simulink model "final_project"  (R2021a)
settings: Solver=FixedStepAuto  StartTime=0.0  StopTime=30  RelTol=1e-3
InitFcn:
  | load('BusDefinitions.mat')
values from neighbouring files (symbols this model uses):
  A_a_dis = [1  -0.0479044950468; 0  1]    [RSdata_Kalman.mat]
  A_e_dis = [1  0.0479044950468; 0  1]    [RSdata_Kalman.mat]
  A_t_dis = [1  0.00488821378028; 0  1]    [RSdata_Kalman.mat]
  B_a_dis = [-0.000119761237617 0.005]    [RSdata_Kalman.mat]
  B_e_dis = [0.000119761237617 0.005]    [RSdata_Kalman.mat]
  B_t_dis = [1.22205344507e-05 0.005]    [RSdata_Kalman.mat]
  C_a_dis = [1  0; 0  1]    [RSdata_Kalman.mat]
  C_e_dis = [1  0; 0  1]    [RSdata_Kalman.mat]
  C_t_dis = [1 0]    [RSdata_Kalman.mat]
  F_aileron = 5.76146350631e-05    [RSdata_Kalman.mat]
  F_elevator = -6.47120901071e-05    [RSdata_Kalman.mat]
  F_rudder = 0.000879878480451    [RSdata_Kalman.mat]
  F_throttle = -0.417330356587    [RSdata_Kalman.mat]
  g = 9.8    [RSdata_Kalman.mat]
  K_A = [5.76146350631e-05 0.000978114789418 0.000483]    [RSdata_Kalman.mat]
  K_E = [-6.47120901071e-05 0.00109860719101 0.0005425]    [RSdata_Kalman.mat]
  K_R = [0.000879878480451 0.00075]    [RSdata_Kalman.mat]
  K_T = [-0.417330356587 -0.34]    [RSdata_Kalman.mat]
  Kappa = 1    [RSdata_Kalman.mat]
  m = 0.068    [RSdata_Kalman.mat]
  M = [2.03476350051e-06 9.69056117119e-08 9.69056117119e-08 -1.05662818468e-08 2.03476350051e-06 -9.69056117119e-08 9.69056117119e-08 1.05662818468e-08 2.03476350051e-06 -9.69056117119e-08 -9.69056117119e-08 -1.05662818468e-08 ... (16 elements, 4x4)]    [RSdata_Kalman.mat]
  R_t = 0.00678306479724    [RSdata_Kalman.mat]
undefined symbols (not defined in the file or in its folder): codertarget, Discrete, Time
libraries: simulink x8, ctrlSharedLib x3
settings Model: ExtModeTrigDuration=80  Creator=tomwh  LastModifiedBy=Liza
settings SolverCC: AlgebraicLoopSolver=TrustRegion
settings OptimizationCC: EnhancedBackFolding=on  PassReuseOutputArgsAs=Individual arguments  ZeroExternalMemoryAtStartup=off  ZeroInternalMemoryAtStartup=off  MaxStackSize=64  OptimizeBlockOrder=speed  DifferentSizesBufferReuse=on  OptimizationCustomize=off  EfficientTunableParamExpr=on
settings DebuggingCC: ParameterTunabilityLossMsg=error  SFMachineParentedDataDiag=warning  ArithmeticOperatorsInVariantConditions=warning
settings HardwareCC: ProdBitPerPointer=32  ProdBitPerSizeT=32  ProdBitPerPtrDiffT=32  ProdLargestAtomicInteger=Long  ProdWordSize=32  ProdHWDeviceType=ARM Compatible->ARM 9  UseEmbeddedCoderFeatures=off
settings SFSimCC: SimUseLocalCustomCode=off  MATLABDynamicMemAlloc=off
settings RTWCC: SystemTargetFile=ert.tlc  HardwareBoard=PARROT Mambo  TemplateMakefile=ert_default_tmf  GenerateReport=on  RTWUseLocalCustomCode=off  Toolchain=Sourcery G++ Lite GNU Toolchain for Drones  LaunchReport=on
settings CodeAppCC: ForceParamTrailComments=on  IgnoreCustomStorageClasses=off  OperatorAnnotations=on  SimulinkDataObjDesc=on  SFDataObjDesc=on  InsertBlockDesc=on
settings ERTTargetCC: MatFileLogging=on  SupportNonInlinedSFcns=on

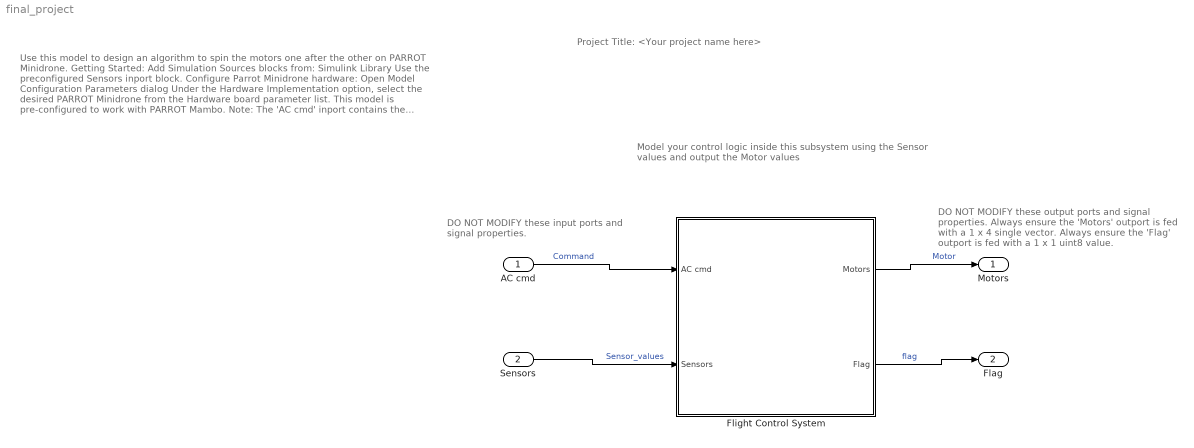
== system final_project ==
  note: Model your control logic inside this subsystem
      | using the Sensor values and output the
      | Motor values
  note: DO NOT MODIFY these output ports
      | and signal properties.
      |
      |
      |
      | Always ensure the 'Motors' outport
      | is fed with a 1 x 4 single vector.
      |
      |
      |
      |
      |
      | Always ensure the 'Flag' outport is
      | fed with a 1 x 1 uint8 value.
  note: DO NOT MODIFY these input
      | ports and signal properties.
  note: Use this model to design an algorithm to spin the motors one
      | after the other on PARROT Minidrone.
      |
      | Getting Started:
      |
      | Add Simulation Sources blocks from:
      | Simulink Library
      | Use the preconfigured Sensors inport block.
      |
      | Configure Parrot Minidrone hardware:
      |
      | Open Model Configuration Parameters dialog
      |
      | Under the Hardware Implementation option, select the desired
      | PARROT Minidrone from the Hardware board parameter list.
      |
      | This model is pre-configured to work with PARROT Mambo.
      |
      | Note:
      |
      | The 'AC cmd' inport contains the position and orientation
      | reference signals information.
      | The 'Sensors' inport contains data from accelerometer,
      | gyroscope, ultrasonic, pressure and optical flow data.
      | The 'Flag' outport can be used to model an error condition
      | which stops the drone.
      | The 'Motors' outport is fed with the speed values of the 4 motors.
      | Learn more:
      |
      | Simulink Subsystem
      | Simulink Buses
  note: Project Title: <Your project name here>
  AC cmd : Inport  OutDataTypeStr=Bus: CommandBus  BusOutputAsStruct=on
  Sensors : Inport  Port=2  OutDataTypeStr=Bus: SensorsBus  BusOutputAsStruct=on
  Flight Control System : Subsystem  InitFcn=codertarget.parrot.internal.fcsSubsystemCallback(gcb);
  Motors : Outport  OutDataTypeStr=single  PortDimensions=[1 4]  VectorParamsAs1DForOutWhenUnconnected=off
  Flag : Outport  Port=2  OutDataTypeStr=uint8  PortDimensions=1  VectorParamsAs1DForOutWhenUnconnected=off
  wires:
  Flight Control System/1(Motors) -> Motors/1  "Motor"
  AC cmd/1 -> Flight Control System/1(AC cmd)  "Command"
  Sensors/1 -> Flight Control System/2(Sensors)  "Sensor_values"
  Flight Control System/2(Flag) -> Flag/1  "flag"

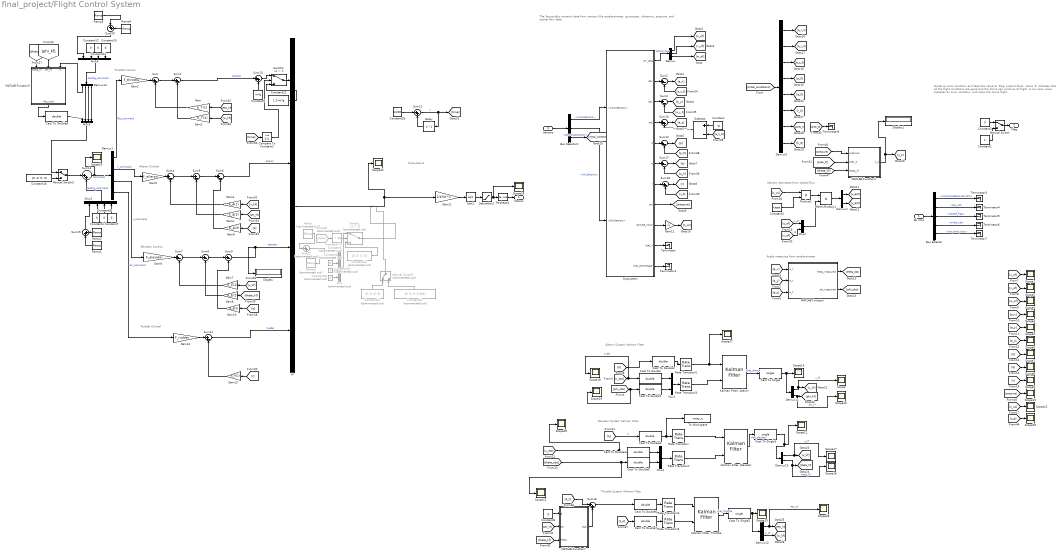
== system final_project/Flight Control System ==
  note: Subsystem1
  note: Angle measures from accelerometer
  note: Velocity estimates from optical flow
  note: Model an error condition and feed the value to 'Flag' outport block.
      | Value '0' indicates that all the flight conditions are good and the drone
      | can continue its flight.
      | A non-zero value indicates an error condition, and stops the drone
      | flight.
  note: The SensorsBus contains data from sensors like
      | accelerometer, gyroscope, ultrasonic, pressure,
      | and optical flow data.
  note: Throttle System Kalman Filter
  note: Elevator System Kalman Filter
  note: Aileron System Kalman Filter
  note: Elevator Control
  note: Aileron Control
  note: Throttle Control
  note: Rudder Control
  AC cmd : Inport
  Sensors : Inport  Port=2
  Bus Selector : BusSelector  OutputSignals=controlModePosVSOrient,pos_ref,takeoff_flag,orient_ref,live_time_ticks
  Bus Selector1 : BusSelector  OutputSignals=VisionSensors,HALSensors,SensorCalibration
  Cast To Double{,1..8} (9 alike) : DataTypeConversion  OutDataTypeStr=double
  Cast To Single : DataTypeConversion  OutDataTypeStr=single
  Cast To Single1 : DataTypeConversion  OutDataTypeStr=single
  Cast To Single2 : DataTypeConversion  OutDataTypeStr=single
  Compare To Constant1 : simulink/Logic and Bit Operations/Compare To Constant  Commented=on  relop=<  const=15  OutDataTypeStr=boolean
  Compare To Constant2 : simulink/Logic and Bit Operations/Compare To Constant  relop=>=  const=0.4  OutDataTypeStr=boolean
  Constant : Constant  Value=-g
  Constant1 : Constant  OutDataTypeStr=uint8
  Constant10 : Constant  Commented=on  Value=[0; 0; 0; 0.004]
  Constant11 : Constant  Commented=on  Value=[0; 0; 0; 0]
  Constant{4,6..7,12..13,15} (6 alike) : Constant  Value=0
  Constant14 : Constant  Commented=on  Value=[0; 0; 0; 0]
  Constant16 : Constant  Value=[0; 0; 0; 0]
  Constant18 : Constant  Value=1/200
  Constant19 : Constant  Commented=on  Value=0
  Constant2 : Constant  Value=0  OutDataTypeStr=uint8
  Constant20 : Constant  Commented=on  Value=0
  Constant21 : Constant  Value=1.1*m*g
  Constant3 : Constant  Value=Kappa
  Constant5 : Constant  Value=m*g
  Constant8 : Constant  Value=g
  Constant9 : Constant  Commented=on  Value=0
  Delay : Delay  DelayLength=1  SampleTime=1/200
  Demux : Demux  Outputs=3
  Demux1 : Demux
  Demux{2,10..12} (4 alike) : Demux  Outputs=2
  Demux14 : Demux
  Demux3 : Demux  Outputs=8
  Display : Display
  Display1 : Display
  From49 : From  Commented=on  GotoTag=time
  Gain : Gain  Gain=K_T(1)
  Gain1 : Gain  Gain=K_T(2)
  Gain10 : Gain  Gain=K_E(3)
  Gain11 : Gain  Gain=1/4*M  Multiplication=Matrix(K*u)
  Gain12 : Gain  Gain=-1
  Gain13 : Gain  Gain=K_R(2)
  Gain14 : Gain  Gain=F_rudder
  Gain2 : Gain  Gain=F_throttle
  Gain3 : Gain  Gain=K_A(1)
  Gain4 : Gain  Gain=K_A(2)
  Gain5 : Gain  Gain=F_aileron
  Gain6 : Gain  Gain=K_A(3)
  Gain7 : Gain  Gain=K_E(1)
  Gain8 : Gain  Gain=K_E(2)
  Gain9 : Gain  Gain=F_elevator
  "Kalman Filter, Aileron" : ctrlSharedLib/Kalman Filter  TimeDomain=Discrete-Time  UseCurrentEstimator=on  ModelSource=Individual A, B, C, D matrices  ModelSourceVariable=ss(0.95,1,1,0,1)  A=A_a_dis  B=B_a_dis  C=C_a_dis  D=0  NumberOfStates=1  NumberOfInputs=1  NumberOfOutputs=1  InitialEstimateSource=Dialog  X0=0  P0=10  UseK=off  UseGH=off  NumberOfProcessNoiseInputs=1  G=1  TimeInvariantG=on  H=0  TimeInvariantH=on  Q=Q_a_dis  TimeInvariantQ=on  R=eye(2)  TimeInvariantR=on  N=0  TimeInvariantN=on  AddInputPort=on  AddEnablePort=off  OutputEstimatedY=off  OutputP=off  Ts=1/200
  "Kalman Filter, Elevator" : ctrlSharedLib/Kalman Filter  TimeDomain=Discrete-Time  UseCurrentEstimator=on  ModelSource=Individual A, B, C, D matrices  ModelSourceVariable=ss(0.95,1,1,0,1)  A=A_e_dis  B=B_e_dis  C=C_e_dis  D=0  NumberOfStates=1  NumberOfInputs=1  NumberOfOutputs=1  InitialEstimateSource=Dialog  X0=0  P0=10  UseK=off  UseGH=off  NumberOfProcessNoiseInputs=1  G=1  TimeInvariantG=on  H=0  TimeInvariantH=on  Q=Q_e_dis  TimeInvariantQ=on  R=[1/100 0; 0 1/25]  TimeInvariantR=on  N=0  TimeInvariantN=on  AddInputPort=on  AddEnablePort=off  OutputEstimatedY=off  OutputP=off  Ts=1/200
  "Kalman Filter, Throttle" : ctrlSharedLib/Kalman Filter  TimeDomain=Discrete-Time  UseCurrentEstimator=on  ModelSource=Individual A, B, C, D matrices  ModelSourceVariable=ss(0.95,1,1,0,1)  A=A_t_dis  B=B_t_dis  C=C_t_dis  D=0  NumberOfStates=1  NumberOfInputs=1  NumberOfOutputs=1  InitialEstimateSource=Dialog  X0=0  P0=10  UseK=off  UseGH=off  NumberOfProcessNoiseInputs=1  G=1  TimeInvariantG=on  H=0  TimeInvariantH=on  Q=Q_t_dis  TimeInvariantQ=on  R=R_t  TimeInvariantR=on  N=0  TimeInvariantN=on  AddInputPort=on  AddEnablePort=off  OutputEstimatedY=off  OutputP=off  Ts=1/200
  MATLAB Function : MATLAB Function  TreatAsAtomicUnit=on
  MATLAB Function1 : MATLAB Function  TreatAsAtomicUnit=on
  MATLAB Function3 : MATLAB Function  TreatAsAtomicUnit=on
  MATLAB Function7 : MATLAB Function  TreatAsAtomicUnit=on
  Manual Switch : ManualSwitch
  Manual Switch2 : ManualSwitch  Commented=on
  Manual Switch3 : ManualSwitch
  MatrixMultiply1 : Product
  Mux : Mux  Commented=on
  Mux1 : Mux  Inputs=2
  Mux2 : Mux  Inputs=2
  Mux3 : Mux
  Mux4 : Mux  Inputs=2
  Mux5 : Mux
  Mux6 : Mux
  Product1 : Product
  Ramp : simulink/Sources/Ramp  Commented=on  slope=m*g/5  start=5  InitialOutput=0
  Ramp1 : simulink/Sources/Ramp  slope=-.2  start=30  InitialOutput=0
  Ramp2 : simulink/Sources/Ramp  slope=.2  start=25  InitialOutput=0
  Ramp3 : simulink/Sources/Ramp  slope=-.2  start=5  InitialOutput=0
  Ramp4 : simulink/Sources/Ramp  slope=.2  start=10  InitialOutput=0
  Ramp5 : simulink/Sources/Ramp  Commented=on  slope=-m*g/5  start=10  InitialOutput=0
  Rate Transition{,1..5} (6 alike) : RateTransition  OutPortSampleTime=dt
  Reshape1 : Reshape  OutputDimensionality=Customize  OutputDimensions=[1,4]
  Saturation1 : Saturate  UpperLimit=500  LowerLimit=0  OutDataTypeStr=single
  Scope{,1..27} (28 alike) : Scope
  Sqrt1 : Sqrt  SaturateOnIntegerOverflow=on
  Subsystem : Subsystem
  Subtract : Sum  Inputs=+-
  Sum{,1..9,11..12,17..18} (14 alike) : Sum  Inputs=|+-
  Sum{10,13..16,20..21} (7 alike) : Sum  Inputs=|++
  Sum22 : Sum  Commented=on  Inputs=|++
  Switch1 : Switch  Commented=on  Criteria=u2 > Threshold
  Switch2 : Switch  Criteria=u2 > Threshold
  Terminator{,1,3..8} (8 alike) : Terminator
  To Workspace : ToWorkspace  VariableName=noisy_q  SaveFormat=Structure With Time  SampleTime=-1
  W : Mux
  Motors : Outport  VectorParamsAs1DForOutWhenUnconnected=off
  Flag : Outport  Port=2  VectorParamsAs1DForOutWhenUnconnected=off
  wires:
  AC cmd/1 -> Bus Selector/1
  Bus Selector/1 -> Terminator3/1  "<controlModePosVSOrient>"
  Bus Selector/2 -> Terminator4/1  "<pos_ref>"
  Bus Selector/3 -> Terminator5/1  "<takeoff_flag>"
  Bus Selector/4 -> Terminator6/1  "<orient_ref>"
  Bus Selector/5 -> Terminator7/1  "<live_time_ticks>"
  Manual Switch/1 -> Flag/1
  Bus Selector1/1 -> Subsystem/1(<VisionSensors>)  "<VisionSensors>"
  Bus Selector1/3 -> [initial_conditions]  "<SensorCalibration>"
  Sensors/1 -> Bus Selector1/1
  Bus Selector1/2 -> Subsystem/2(<HALSensors>)  "<HALSensors>"
  Subsystem/10(vbat_V) -> Terminator/1
  Subsystem/11(vbat_percentage) -> Terminator1/1
  Subsystem/1(OF_data) -> Demux/1  "optical_flow"
  Demux/1 -> [u_of]
  Demux/2 -> [v_of]
  Demux/3 -> [w_of]
  Subsystem/8(prs) -> [pressure]
  [u_of] -> Scope1/1
  [v_of] -> Scope2/1
  [w_of] -> Scope3/1
  [a_x] -> Scope4/1
  [a_y] -> Scope5/1
  [a_z] -> Scope6/1
  [p] -> Scope7/1
  [q] -> Scope8/1
  [r] -> Scope9/1
  [pressure] -> Scope12/1
  [z_us] -> Scope13/1
  Mux2/1 -> MatrixMultiply1/2
  Product1/1 -> MatrixMultiply1/1
  [v_of] -> Mux2/2  "v_of"
  Demux2/2 -> [v_est]
  MatrixMultiply1/1 -> Demux2/1
  Demux2/1 -> [u_est]
  Constant3/1 -> Product1/2
  [u_of] -> Mux2/1  "u_of"
  [z_us] -> Product1/1
  [a_z] -> MATLAB Function/3(a_z)
  [a_x] -> MATLAB Function/1(a_x)
  [a_y] -> MATLAB Function/2(a_y)
  MATLAB Function/1(theta_measured) -> [theta_obs]
  MATLAB Function/2(phi_measured) -> [phi_obs]
  Constant2/1 -> Manual Switch/1
  Constant1/1 -> Manual Switch/2
  Sqrt1/1 -> Saturation1/1
  "Kalman Filter, Throttle"/1 -> Cast To Single2/1  "xhat_throttle"
  [v_est] -> Scope18/1, Cast To Double/1  "v_est"
  Mux4/1 -> Rate Transition1/1
  Demux12/1 -> Scope26/1, [Pbz_kf]  "Pbz_kf"
  Cast To Double2/1 -> Rate Transition2/1
  Cast To Single/1 -> Demux11/1, Scope14/1
  Cast To Double4/1 -> Mux4/1
  Demux12/2 -> [w_kf]  "w_kf"
  Demux10/1 -> Scope17/1, [u_kf]  "u_kf"
  Mux1/1 -> Rate Transition3/1
  Rate Transition/1 -> "Kalman Filter, Elevator"/1
  [phi_obs] -> Scope19/1, Cast To Double1/1
  Rate Transition5/1 -> "Kalman Filter, Throttle"/2
  "Kalman Filter, Aileron"/1 -> Cast To Single/1  "xhat_aileron"
  Demux11/2 -> Scope10/1, [phi_kf]  "phi_kf"
  Sum16/1 -> Cast To Double6/1
  Rate Transition3/1 -> "Kalman Filter, Aileron"/2
  Cast To Double7/1 -> Rate Transition5/1
  Rate Transition2/1 -> Scope27/1, "Kalman Filter, Aileron"/1
  Demux10/2 -> Scope16/1, [theta_kf]  "theta_kf"
  [a_z] -> Sum16/1
  Rate Transition1/1 -> "Kalman Filter, Elevator"/2
  Rate Transition4/1 -> "Kalman Filter, Throttle"/1
  "Kalman Filter, Elevator"/1 -> Cast To Single1/1  "xhat_elevator"
  Demux11/1 -> Scope/1, [v_kf]  "v_kf"
  Cast To Single1/1 -> Demux10/1, Scope11/1
  Cast To Double1/1 -> Mux1/2
  Cast To Single2/1 -> Demux12/1, Scope15/1
  Cast To Double3/1 -> To Workspace/1, Rate Transition/1
  Cast To Double6/1 -> Rate Transition4/1
  Cast To Double5/1 -> Mux4/2
  Cast To Double/1 -> Mux1/1
  [p] -> Cast To Double2/1
  [q] -> Cast To Double3/1  "q"
  Gain14/1 -> Sum11/1
  Demux1/2 -> Gain5/1  "v_command"
  Constant6/1 -> Mux3/3
  Demux1/4 -> Gain14/1  "psi_command"
  Constant7/1 -> Mux3/4
  Constant4/1 -> Mux3/2
  Sum15/1 -> Mux3/1
  Gain13/1 -> Sum11/2
  Sum9/1 -> W/3, Display/1  "elevator"
  Constant5/1 -> Sum13/2
  Demux1/1 -> Gain2/1  "Pbz_command"
  Sum6/1 -> W/2  "aileron"
  Sum7/1 -> Sum8/1
  Gain2/1 -> Sum/1
  [phi_kf] -> Gain4/1
  Sum5/1 -> Sum6/1
  [q] -> Gain10/1
  [w_kf] -> Gain1/1
  [theta_kf] -> MATLAB Function3/1(theta_kf)
  Ramp1/1 -> Sum15/1
  Sum1/1 -> Sum13/1  "throttle"
  Gain1/1 -> Sum1/2
  Demux14/4 -> Mux5/4
  MATLAB Function3/1(Pbz_cmd) -> Cast To Double8/1
  Demux14/1 -> MATLAB Function3/3(P_D_cmd)
  Sum4/1 -> Sum5/1
  Sum14/1 -> Scope23/1, Demux1/1  "Command"
  [phi_kf] -> MATLAB Function3/2(phi_kf)
  Gain9/1 -> Sum7/1
  Gain4/1 -> Sum5/2
  Gain10/1 -> Sum9/2
  [r] -> Gain13/1
  [Pbz_kf] -> Gain/1
  Sum11/1 -> W/4  "rrudder"
  [theta_kf] -> Gain8/1
  Gain7/1 -> Sum7/2
  Demux1/3 -> Gain9/1  "u_command"
  Sum8/1 -> Sum9/1
  [p] -> Gain6/1
  Gain8/1 -> Sum8/2
  Gain5/1 -> Sum4/1
  Gain6/1 -> Sum6/2
  Cast To Double8/1 -> Mux5/1
  Gain3/1 -> Sum4/2
  Demux14/3 -> Mux5/3
  Sum/1 -> Sum1/1
  Demux14/2 -> Mux5/2
  Gain/1 -> Sum/2
  Ramp2/1 -> Sum15/2
  [v_kf] -> Gain3/1
  [u_kf] -> Gain7/1
  [initial_conditions] -> Demux3/1
  Demux3/1 -> [a_x_0]
  Demux3/2 -> [a_y_0]
  Demux3/3 -> [a_z_0]
  Demux3/4 -> [p_0]
  Demux3/5 -> [q_0]
  Demux3/6 -> [r_0]
  Demux3/7 -> [pres_0]
  Demux3/8 -> [h_0]
  Subsystem/2(ddx) -> Sum2/1
  Sum2/1 -> [a_x]
  [a_x_0] -> Sum2/2
  Subsystem/3(ddy) -> Sum3/1
  Sum3/1 -> [a_y]
  [a_y_0] -> Sum3/2
  Subsystem/4(ddz) -> Sum10/1
  Sum10/1 -> [a_z]
  Subsystem/5(p) -> Sum12/1
  Sum12/1 -> [p]
  [p_0] -> Sum12/2
  Subsystem/6(q) -> Sum17/1
  Sum17/1 -> [q]
  [q_0] -> Sum17/2
  Subsystem/7(r) -> Sum18/1
  Sum18/1 -> [r]
  [r_0] -> Sum18/2
  Constant8/1 -> MATLAB Function7/1(g)
  MATLAB Function7/1(bias) -> Sum16/2
  [phi_kf] -> MATLAB Function7/2(phi)
  [theta_kf] -> MATLAB Function7/3(theta)
  Constant/1 -> Subtract/1
  [a_z_0] -> Subtract/2
  Subtract/1 -> Sum10/2
  [pres_0] -> Terminator8/1
  [u_est] -> Cast To Double4/1, Scope20/1
  [theta_obs] -> Scope21/1, Cast To Double5/1
  Mux3/1 -> Sum14/2  "landing_command"
  Constant10/1 -> Manual Switch2/2
  Constant11/1 -> Manual Switch2/1
  Manual Switch2/1 -> ?
  Constant12/1 -> Mux6/2
  Ramp3/1 -> Sum20/1
  Ramp4/1 -> Sum20/2
  Constant13/1 -> Mux6/3
  Sum20/1 -> Mux6/1
  Constant15/1 -> Mux6/4
  Mux6/1 -> Demux14/1  "landing_command"
  Manual Switch3/1 -> Sum14/1
  Constant16/1 -> Manual Switch3/2
  Mux5/1 -> Manual Switch3/1
  [pressure] -> MATLAB Function1/1(pressure)
  [pres_0] -> MATLAB Function1/2(pres_0)
  MATLAB Function1/1(z_p) -> Display1/1, [z_p]
  [z_p] -> Cast To Double7/1
  [z_p] -> Scope25/1
  [theta_kf] -> MATLAB Function1/3(theta_kf)
  Subsystem/9(altitude_sonar) -> Gain12/1
  Gain12/1 -> [z_us]
  Constant18/1 -> Sum21/1
  Sum21/1 -> [time], Delay/1  "t"
  Delay/1 -> Sum21/2
  Gain11/1 -> Sqrt1/1
  Ramp/1 -> Sum22/1
  Ramp5/1 -> Sum22/2
  Compare To Constant1/1 -> Switch1/2
  From49/1 -> Compare To Constant1/1
  Constant9/1 -> Mux/2
  Constant19/1 -> Mux/3
  Constant20/1 -> Mux/4
  Sum22/1 -> Mux/1
  Saturation1/1 -> Scope24/1, Reshape1/1
  Reshape1/1 -> Motors/1
  Switch1/1 -> ?
  Mux/1 -> Switch1/1
  Constant14/1 -> Switch1/3
  [time] -> Compare To Constant2/1
  Switch2/1 -> W/1
  Sum13/1 -> Switch2/1
  Compare To Constant2/1 -> Switch2/2
  Constant21/1 -> Switch2/3
  W/1 -> Scope22/1, Gain11/1

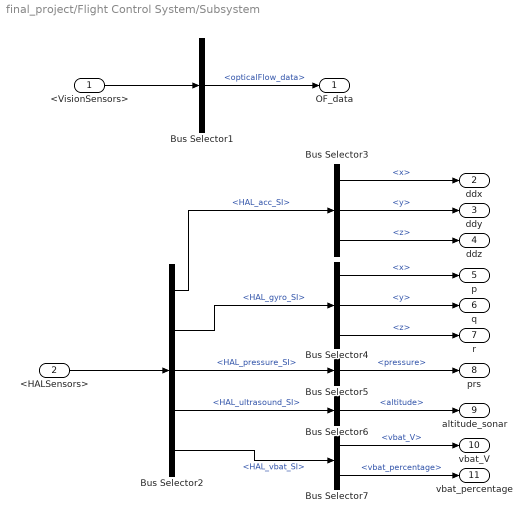
== system final_project/Flight Control System/Subsystem ==
  <VisionSensors> : Inport
  <HALSensors> : Inport  Port=2
  Bus Selector1 : BusSelector  OutputSignals=opticalFlow_data
  Bus Selector2 : BusSelector  OutputSignals=HAL_acc_SI,HAL_gyro_SI,HAL_pressure_SI,HAL_ultrasound_SI,HAL_vbat_SI
  Bus Selector3 : BusSelector  OutputSignals=x,y,z
  Bus Selector4 : BusSelector  OutputSignals=x,y,z
  Bus Selector5 : BusSelector  OutputSignals=pressure
  Bus Selector6 : BusSelector  OutputSignals=altitude
  Bus Selector7 : BusSelector  OutputSignals=vbat_V,vbat_percentage
  OF_data : Outport  VectorParamsAs1DForOutWhenUnconnected=off
  ddx : Outport  Port=2  VectorParamsAs1DForOutWhenUnconnected=off
  ddy : Outport  Port=3  VectorParamsAs1DForOutWhenUnconnected=off
  ddz : Outport  Port=4  VectorParamsAs1DForOutWhenUnconnected=off
  p : Outport  Port=5  VectorParamsAs1DForOutWhenUnconnected=off
  q : Outport  Port=6  VectorParamsAs1DForOutWhenUnconnected=off
  r : Outport  Port=7  VectorParamsAs1DForOutWhenUnconnected=off
  prs : Outport  Port=8  VectorParamsAs1DForOutWhenUnconnected=off
  altitude_sonar : Outport  Port=9  VectorParamsAs1DForOutWhenUnconnected=off
  vbat_V : Outport  Port=10  VectorParamsAs1DForOutWhenUnconnected=off
  vbat_percentage : Outport  Port=11  VectorParamsAs1DForOutWhenUnconnected=off
  wires:
  <VisionSensors>/1 -> Bus Selector1/1
  <HALSensors>/1 -> Bus Selector2/1
  Bus Selector1/1 -> OF_data/1  "<opticalFlow_data>"
  Bus Selector2/1 -> Bus Selector3/1  "<HAL_acc_SI>"
  Bus Selector2/2 -> Bus Selector4/1  "<HAL_gyro_SI>"
  Bus Selector2/3 -> Bus Selector5/1  "<HAL_pressure_SI>"
  Bus Selector2/4 -> Bus Selector6/1  "<HAL_ultrasound_SI>"
  Bus Selector2/5 -> Bus Selector7/1  "<HAL_vbat_SI>"
  Bus Selector3/1 -> ddx/1  "<x>"
  Bus Selector3/2 -> ddy/1  "<y>"
  Bus Selector3/3 -> ddz/1  "<z>"
  Bus Selector4/2 -> q/1  "<y>"
  Bus Selector4/1 -> p/1  "<x>"
  Bus Selector4/3 -> r/1  "<z>"
  Bus Selector5/1 -> prs/1  "<pressure>"
  Bus Selector6/1 -> altitude_sonar/1  "<altitude>"
  Bus Selector7/1 -> vbat_V/1  "<vbat_V>"
  Bus Selector7/2 -> vbat_percentage/1  "<vbat_percentage>"

== matlab function final_project/Flight Control System/MATLAB Function1 ==
  data: pressure input; z_p output; pres_0 input; theta_kf input
function z_p = fcn(pressure,pres_0,theta_kf) 
g = 9.8; % acceleration due to gravity m/s^2
M = 0.0289644; % molar mass of air in kg/mol
R = 8.31432; % universal gas constant Nm/mol/k
p0 = 101325; % Pa standard pressure

T =288.15;  % Assumed temperature in kelvin
K =-g*M/R/T;
z_p = (1/K.*log(pressure./p0) - 1/K.*log(pres_0./p0))/cos(theta_kf);

== matlab function final_project/Flight Control System/MATLAB Function ==
  data: a_x input; theta_measured output; a_y input; a_z input; phi_measured output
function [theta_measured,phi_measured]= fcn(a_x,a_y,a_z)
theta_measured = -a_x / sqrt(a_y^2 + a_z^2);
phi_measured = a_y/a_z;

== matlab function final_project/Flight Control System/MATLAB Function3 ==
  data: theta_kf input; phi_kf input; P_D_cmd input; Pbz_cmd output
function Pbz_cmd = fcn(theta_kf,phi_kf,P_D_cmd)
    phi = phi_kf;
    theta = theta_kf;
    psi = 0;
    R_phi = [1 0 0;
             0 cos(phi) sin(phi);
             0 -sin(phi) cos(phi)];
    R_theta = [cos(theta) 0 -sin(theta);
               0 1 0;
               sin(theta) 0 cos(theta)];
    R_psi = [cos(psi) sin(psi) 0;
             -sin(psi) cos(psi) 0;
             0 0 1];
    R = R_phi*R_theta*R_psi;
    Pb = R*[0; 0; P_D_cmd];
    Pbz_cmd = Pb(3);

== matlab function final_project/Flight Control System/MATLAB Function7 ==
  data: g input; bias output; phi input; theta input
function bias = fcn(g,phi,theta)
psi = 0;
R_phi = [1 0 0;
         0 cos(phi) sin(phi);
         0 -sin(phi) cos(phi)];
R_theta = [cos(theta) 0 -sin(theta);
           0 1 0;
           sin(theta) 0 cos(theta)];
R_psi = [cos(psi) sin(psi) 0;
         -sin(psi) cos(psi) 0;
         0 0 1];
R = R_phi*R_theta*R_psi;
G_b = R*[0; 0; g];
bias = G_b(3);
